simulink model "bd_par_auto2"  (Simulink 4.1.1)
settings: Solver=ode1  SolverMode=SingleTasking  StartTime=0.0  StopTime=max(cyc_mph(:,1))  FixedStep=1  MaxStep=1  RelTol=1e-3  AbsTol=1e-3
undefined symbols (not defined in the file): air_cp, amb_tmp, cs_charge_deplete_bool, cs_charge_trq, cs_electric_decel_spd, cs_electric_launch_spd_hi, cs_electric_launch_spd_lo, cs_hi_soc, cs_lo_soc, cs_min_trq_frac, cs_off_trq_frac, cyc_avg_time, cyc_cargo_mass, cyc_elevation_init, cyc_filter_bool, cyc_grade, cyc_mph, enable_stop, ess_cap_scale, ess_coulombic_eff, ess_init_soc, ess_max_ah_cap, ess_max_volts, ess_min_volts, ess_mod_airflow, ess_mod_cp, ess_mod_init_tmp, ess_module_mass, ess_module_num, ess_on, ess_res_scale_coef, ess_res_scale_fun, ess_set_tmp, ess_th_calc, ess_th_res_off, ess_th_res_on, ess_tmp, ess_voc, ex_calc, fc_ct_trq, fc_emis, fc_inertia, fc_map_spd, fc_max_trq, fc_on, fc_spd_scale, fc_trq_scale, fc_tstat, fd_inertia, fd_loss, fd_ratio, gb_dnshift_load, gb_dnshift_spd, gb_gears_num, gb_inertia, gb_num_init, gb_ratio, gb_shift_delay, gb_spd_scale, gb_trq_scale ... (+56)
libraries: lib_wheel2 x12, lib_accessory2 x3, lib_etc x2, lib_drive_cycle2 x1, lib_interactive x1, lib_drive_cycle x1, lib_exhaust x1, lib_fuel_converter3 x1
(part 2 of 18)

== system bd_par_auto2/<cs> control strategy/Automatic Transmission  Control ==
  Bus Selector1 : BusSelector  OutputSignals=shifting  MuxedOutput=off
  Bus Selector10 : BusSelector  OutputSignals=eta_gb  MuxedOutput=off
  Bus Selector4 : BusSelector  OutputSignals=slip_limited  MuxedOutput=off
  Bus Selector7 : BusSelector  OutputSignals=gb_trq_out_r,gb_spd_out_r  MuxedOutput=off
  Memory : Memory  X0=1  InheritSampleTime=off
      settings: RTWStateStorageClass=Auto
  Mux1 : Mux  Inputs=3
  Mux2 : Mux  Inputs=2
  gearbox control for automatic transmission : Subsystem  TreatAsAtomicUnit=on
      settings: RTWFcnNameOpts=Auto  RTWFileNameOpts=Auto
  tag scope: gbControl=global, htcControl=global
  wires:
  Mux1/1 -> [gbControl], Bus Selector1/1
  gearbox control for automatic transmission/3(gear number) -> Mux1/3  "gear_number"
  gearbox control for automatic transmission/2(shifting) -> Mux1/2  "shifting"
  gearbox control for automatic transmission/1(gear ratio) -> Mux1/1  "gear_ratio"
  Memory/1 -> gearbox control for automatic transmission/1("eta_gb, t=(i-1)")
  [gbReqOut] -> Bus Selector7/1
  Bus Selector7/1 -> gearbox control for automatic transmission/2(T_gb_out)  "<gb_trq_out_r>"
  Bus Selector10/1 -> Memory/1  "<eta_gb>"
  [gbSensors] -> Bus Selector10/1
  [vehReqOut] -> Bus Selector4/1
  Bus Selector4/1 -> gearbox control for automatic transmission/4(slip_limited)  "<slip_limited>"
  Bus Selector7/2 -> gearbox control for automatic transmission/3(w_gb_out)  "<gb_spd_out_r>"
  Mux2/1 -> [htcControl]
  gearbox control for automatic transmission/4(locked_up) -> Mux2/2  "lock_up"
  Bus Selector1/1 -> Mux2/1  "<shifting>"

== system bd_par_auto2/<cs> control strategy/Clutch Control ==
  Bus Creator : BusCreator  Inputs=3
  Bus Selector : BusSelector  OutputSignals=mpha  MuxedOutput=off
  Bus Selector1 : BusSelector  OutputSignals=shifting  MuxedOutput=off
  Bus Selector2 : BusSelector  OutputSignals=gb_spd_in_a  MuxedOutput=off
  Bus Selector3 : BusSelector  OutputSignals=clutch_trq_out_r  MuxedOutput=off
  Bus Selector4 : BusSelector  OutputSignals=clutch_spd_out_r  MuxedOutput=off
  Bus Selector5 : BusSelector  OutputSignals=veh_spd_a_rec  MuxedOutput=off
  Bus Selector6 : BusSelector  OutputSignals=cycle_mph_r  MuxedOutput=off
  Bus Selector7 : BusSelector  OutputSignals=v_ave_req  MuxedOutput=off
  Bus Selector8 : BusSelector  OutputSignals=engine_on  MuxedOutput=off
  Clutch Control : Subsystem  TreatAsAtomicUnit=on
      settings: RTWFcnNameOpts=Auto  RTWFileNameOpts=Auto
  Memory1 : Memory  X0=0  InheritSampleTime=off
      settings: RTWStateStorageClass=Auto
  Memory2 : Memory  X0=cyc_mph(1,2)  InheritSampleTime=off
      settings: RTWStateStorageClass=Auto
  Memory3 : Memory  X0=0  InheritSampleTime=off
      settings: RTWStateStorageClass=Auto
  Memory4 : Memory  X0=cyc_mph(1,2)  InheritSampleTime=off
      settings: RTWStateStorageClass=Auto
  tag scope: clControl=global
  wires:
  Memory4/1 -> Clutch Control/7(cyc_mph_r)
  Memory3/1 -> Clutch Control/6(veh_spd_a_rec)
  Memory2/1 -> Clutch Control/5(mpha)
  Memory1/1 -> Clutch Control/2(gb_spd_in_a)
  Clutch Control/3(launch_flag) -> Bus Creator/3  "launch_flag"
  Bus Selector4/1 -> Clutch Control/4(w_cl_out)  "<clutch_spd_out_r>"
  Bus Selector3/1 -> Clutch Control/3(T_cl_out)  "<clutch_trq_out_r>"
  [clReqOut] -> Bus Selector4/1, Bus Selector3/1
  Bus Selector2/1 -> Memory1/1  "<gb_spd_in_a>"
  [gbSensors] -> Bus Selector2/1
  Bus Selector1/1 -> Clutch Control/1(shifting)  "<shifting>"
  [gbControl] -> Bus Selector1/1
  Clutch Control/2(launch_speed) -> Bus Creator/2  "launch_speed"
  Clutch Control/1(clutch_state) -> Bus Creator/1  "clutch_state"
  Bus Creator/1 -> [clControl]
  [vehSensors] -> Bus Selector/1
  Bus Selector/1 -> Memory2/1  "<mpha>"
  [vehSensors] -> Bus Selector5/1
  Bus Selector5/1 -> Memory3/1  "<veh_spd_a_rec>"
  [cycReqOut] -> Bus Selector6/1
  Bus Selector6/1 -> Memory4/1  "<cycle_mph_r>"
  [vehReqOut] -> Bus Selector7/1
  Bus Selector7/1 -> Clutch Control/8(v_ave_req)  "<v_ave_req>"
  [fcControl] -> Bus Selector8/1
  Bus Selector8/1 -> Clutch Control/9(engine_on?)  "<engine_on>"

== system bd_par_auto2/<cs> control strategy/Drive Cycle ==
  Bus Creator : BusCreator  Inputs=4
  Bus Selector : BusSelector  OutputSignals=mpha  MuxedOutput=off
  Constant : Constant  Value=0
  drive cycle dummy controller : lib_drive_cycle2/drive cycle controls/drive cycle dummy controller
      settings: RTWFcnNameOpts=Auto  RTWFileNameOpts=Auto
  tag scope: cycControl=global
  wires:
  [vehSensors] -> Bus Selector/1
  Bus Selector/1 -> drive cycle dummy controller/1  "<mpha>"
  Constant/1 -> drive cycle dummy controller/3, drive cycle dummy controller/2, drive cycle dummy controller/4
  drive cycle dummy controller/1 -> Bus Creator/1  "mpha"
  drive cycle dummy controller/2 -> Bus Creator/2  "altia_grade"
  drive cycle dummy controller/3 -> Bus Creator/3  "Altia_Run"
  drive cycle dummy controller/4 -> Bus Creator/4  "altia_cyc_mph_r"
  Bus Creator/1 -> [cycControl]

== system bd_par_auto2/<cs> control strategy/Electrical Accessories ==
  Bus Creator : BusCreator  Inputs=4
  Bus Selector1 : BusSelector  OutputSignals=F_req  MuxedOutput=off
  Bus Selector2 : BusSelector  OutputSignals=key_on  MuxedOutput=off
  Bus Selector3 : BusSelector  OutputSignals=engine_on  MuxedOutput=off
  Constant : Constant  Value=ess_on*1
  electrical accessory controller : Subsystem
      settings: RTWFcnNameOpts=Auto  RTWFileNameOpts=Auto
  tag scope: acceControl=global
  wires:
  Constant/1 -> electrical accessory controller/1(electrical accessories on?)
  Bus Creator/1 -> [acceControl]
  [fcControl] -> Bus Selector2/1
  Bus Selector2/1 -> electrical accessory controller/3(key_on in)  "<key_on>"
  [fcControl] -> Bus Selector3/1
  Bus Selector3/1 -> electrical accessory controller/4(engine_on in)  "<engine_on>"
  [vehReqOut] -> Bus Selector1/1
  Bus Selector1/1 -> electrical accessory controller/2(F_req in)  "<F_req>"
  electrical accessory controller/1(acc_on) -> Bus Creator/1
  electrical accessory controller/2(F_req) -> Bus Creator/2
  electrical accessory controller/3(key_on) -> Bus Creator/3
  electrical accessory controller/4(engine_on) -> Bus Creator/4

== system bd_par_auto2/<cs> control strategy/Fuel Converter Control parallel hybrid  ic engine ==
  note: Controls for Fuel Converter:
      | IC Engine for Parallel Hybrid
  Bus Creator : BusCreator  Inputs=10
  Bus Selector1 : BusSelector  OutputSignals=clutch_state  MuxedOutput=off
  Bus Selector10 : BusSelector  OutputSignals=v_req_limited  MuxedOutput=off
  Bus Selector11 : BusSelector  OutputSignals=SOC  MuxedOutput=off
  Bus Selector12 : BusSelector  OutputSignals=ess_max_pwr  MuxedOutput=off
  Bus Selector13 : BusSelector  OutputSignals=fc_clt_tmp  MuxedOutput=off
  Bus Selector14 : BusSelector  OutputSignals=T_cl_out  MuxedOutput=off
  Bus Selector15 : BusSelector  OutputSignals=w_cl_out  MuxedOutput=off
  Bus Selector2 : BusSelector  OutputSignals=shifting  MuxedOutput=off
  Bus Selector3 : BusSelector  OutputSignals=acc_mech_trq_a  MuxedOutput=off
  Bus Selector4 : BusSelector  OutputSignals=v_prev  MuxedOutput=off
  Bus Selector5 : BusSelector  OutputSignals=cycle_mph_r  MuxedOutput=off
  Bus Selector6 : BusSelector  OutputSignals=veh_spd_a_rec  MuxedOutput=off
  Bus Selector7 : BusSelector  OutputSignals=gear_ratio  MuxedOutput=off
  Bus Selector8 : BusSelector  OutputSignals=current_veh_mass  MuxedOutput=off
  Bus Selector9 : BusSelector  OutputSignals=mpha  MuxedOutput=off
  Fuel Converter Control : Subsystem
      settings: RTWFcnNameOpts=Auto  RTWFileNameOpts=Auto
  Memory{1..3,5} (4 alike) : Memory  X0=0  InheritSampleTime=off
      settings: RTWStateStorageClass=Auto
  tag scope: fcControl=global
  wires:
  Bus Selector2/1 -> Fuel Converter Control/9(shifting)  "<shifting>"
  Bus Selector7/1 -> Fuel Converter Control/3(gear_ratio)  "<gear_ratio>"
  Bus Selector1/1 -> Fuel Converter Control/1(clutch_state)  "<clutch_state>"
  [clControl] -> Bus Selector1/1
  [gbControl] -> Bus Selector7/1
  [fcSensors] -> Fuel Converter Control/8(fcSensors)
  [vehReqOut] -> Bus Selector4/1
  Bus Selector4/1 -> Fuel Converter Control/10(v_prev)  "<v_prev>"
  [gbControl] -> Bus Selector2/1
  [accmSensors] -> Bus Selector3/1
  Bus Selector3/1 -> Memory5/1  "<acc_mech_trq_a>"
  Memory5/1 -> Fuel Converter Control/7(acc_mech_trq_est)
  [cycReqOut] -> Bus Selector5/1
  Bus Selector5/1 -> Memory3/1  "<cycle_mph_r>"
  [vehSensors] -> Bus Selector6/1
  Bus Selector6/1 -> Memory2/1  "<veh_spd_a_rec>"
  [cycSensors] -> Bus Selector8/1
  Bus Selector8/1 -> Fuel Converter Control/4(current_veh_mass)  "<current_veh_mass>"
  [vehSensors] -> Bus Selector9/1
  Bus Selector9/1 -> Memory1/1  "<mpha>"
  Fuel Converter Control/10(v_prev out) -> Bus Creator/10  "v_prev"
  Fuel Converter Control/9(key_on out) -> Bus Creator/9  "key_on"
  Fuel Converter Control/8(engine_on out) -> Bus Creator/8  "engine_on"
  Fuel Converter Control/7(acc_mech_trq_est out) -> Bus Creator/7  "acc_mech_trq_est"
  Fuel Converter Control/6(cyc_mph_r out) -> Bus Creator/6  "cyc_mph_r_prev"
  Fuel Converter Control/5(veh spd a rec out) -> Bus Creator/5  "veh_spd_a_rec_prev"
  Fuel Converter Control/4(current veh mass out) -> Bus Creator/4  "current_veh_mass"
  Fuel Converter Control/3(gear_ratio out) -> Bus Creator/3  "gear_ratio"
  Fuel Converter Control/2(miles per hour out) -> Bus Creator/2  "mpha_prev"
  Fuel Converter Control/1(clutch state out) -> Bus Creator/1  "clutch_state"
  Bus Creator/1 -> [fcControl]
  Memory1/1 -> Fuel Converter Control/2(mpha(t-1) (prev))
  Memory2/1 -> Fuel Converter Control/5(veh_spd_a_rec(t-1) (prev))
  Memory3/1 -> Fuel Converter Control/6(cyc_mph_r(t-1) (prev))
  [vehSensors] -> Bus Selector10/1
  Bus Selector10/1 -> Fuel Converter Control/11(v_req_limited)  "<v_req_limited>"
  [essSensors] -> Bus Selector11/1
  Bus Selector11/1 -> Fuel Converter Control/12(SOC)  "<SOC>"
  [essSensors] -> Bus Selector12/1
  Bus Selector12/1 -> Fuel Converter Control/13(ess_max_pwr)  "<ess_max_pwr>"
  [fcSensors] -> Bus Selector13/1
  Bus Selector13/1 -> Fuel Converter Control/14(fc_clt_tmp)  "<fc_clt_tmp>"
  [clSensors] -> Bus Selector14/1
  Bus Selector14/1 -> Fuel Converter Control/15(T_cl_out)  "<T_cl_out>"
  [clSensors] -> Bus Selector15/1
  Bus Selector15/1 -> Fuel Converter Control/16(w_cl_out)  "<w_cl_out>"

== system bd_par_auto2/<cs> control strategy/Hybrid  Engine Torque Modification Strategy ==
  Bus Creator : BusCreator  Inputs=3
  Bus Selector : BusSelector  OutputSignals=tm_spd_out_r  MuxedOutput=off
  Bus Selector1 : BusSelector  OutputSignals=SOC  MuxedOutput=off
  Bus Selector2 : BusSelector  OutputSignals=engine_on  MuxedOutput=off
  parallel auto hybrid torque control : Subsystem
      settings: RTWFcnNameOpts=Auto  RTWFileNameOpts=Auto
  tag scope: tmControl=global
  wires:
  parallel auto hybrid torque control/1(tm_torqueMod) -> Bus Creator/1  "tm_torqueMod"
  parallel auto hybrid torque control/2(tm_torqueMin) -> Bus Creator/2  "tm_torqueMin"
  parallel auto hybrid torque control/3(tm_enable) -> Bus Creator/3  "tm_enable"
  Bus Creator/1 -> [tmControl]
  [tmReqOut] -> Bus Selector/1
  Bus Selector/1 -> parallel auto hybrid torque control/1(tm_spd_out_r)  "<tm_spd_out_r>"
  [essSensors] -> Bus Selector1/1
  Bus Selector1/1 -> parallel auto hybrid torque control/2(SOC)  "<SOC>"
  [fcControl] -> Bus Selector2/1
  Bus Selector2/1 -> parallel auto hybrid torque control/3(engine_on)  "<engine_on>"

== system bd_par_auto2/<cs> control strategy/Mechanical Accessories ==
  Bus Creator : BusCreator  Inputs=9
  Bus Selector : BusSelector  OutputSignals=fc_spd_est  MuxedOutput=off
  Bus Selector1 : BusSelector  OutputSignals=F_req  MuxedOutput=off
  Bus Selector2 : BusSelector  OutputSignals=key_on  MuxedOutput=off
  Bus Selector3 : BusSelector  OutputSignals=engine_on  MuxedOutput=off
  Constant : Constant  Value=not(ess_on)*1
  Constant1 : Constant  Value=inf
  Constant2 : Constant  Value=(vc_idle_spd*vc_idle_bool)+eps
  mechanical accessory controller : Subsystem
      settings: RTWFcnNameOpts=Auto  RTWFileNameOpts=Auto
  tag scope: accmControl=global
  wires:
  Constant1/1 -> mechanical accessory controller/2(maximum accessory speed)
  Constant2/1 -> mechanical accessory controller/3(minimum accessory speed)
  Constant/1 -> mechanical accessory controller/4(electrical accessories on?)
  mechanical accessory controller/1(acc_on) -> Bus Creator/1
  mechanical accessory controller/2(acc_mech_spd_r) -> Bus Creator/2
  mechanical accessory controller/3(acc_mech_spd_a) -> Bus Creator/3
  mechanical accessory controller/4(acc_max_spd) -> Bus Creator/4
  mechanical accessory controller/5(acc_min_spd) -> Bus Creator/5
  mechanical accessory controller/6(elec_acc_on_bool) -> Bus Creator/6
  mechanical accessory controller/7(F_req) -> Bus Creator/7
  mechanical accessory controller/8(key_on) -> Bus Creator/8
  mechanical accessory controller/9(engine_on) -> Bus Creator/9
  Bus Creator/1 -> [accmControl]
  [fcControl] -> Bus Selector2/1
  Bus Selector2/1 -> mechanical accessory controller/6(key on?)  "<key_on>"
  [fcControl] -> Bus Selector3/1
  Bus Selector3/1 -> mechanical accessory controller/7(engine on?)  "<engine_on>"
  [fcReqOut] -> Bus Selector/1
  Bus Selector/1 -> mechanical accessory controller/1(accessory reference shaft speed)  "<fc_spd_est>"
  [vehReqOut] -> Bus Selector1/1
  Bus Selector1/1 -> mechanical accessory controller/5(Force required for vehicle motion)  "<F_req>"

== system bd_par_auto2/<cs> control strategy/Motor Controller ==
  Bus Selector : BusSelector  OutputSignals=v_prev  MuxedOutput=off
  Bus Selector1 : BusSelector  OutputSignals=key_on  MuxedOutput=off
  Bus Selector2 : BusSelector  OutputSignals=veh_spd_a_rec  MuxedOutput=off
  Bus Selector3 : BusSelector  OutputSignals=bus_voltage  MuxedOutput=off
  Bus Selector4 : BusSelector  OutputSignals=mpha  MuxedOutput=off
  Bus Selector5 : BusSelector  OutputSignals=cycle_mph_r  MuxedOutput=off
  Bus Selector6 : BusSelector  OutputSignals=current_veh_mass  MuxedOutput=off
  Bus Selector7 : BusSelector  OutputSignals=shifting  MuxedOutput=off
  Constant : Constant  Value=cyc_mph(1,2)*0.447/wh_radius*fd_ratio*max(gb_ratio)*tc_mc_to_fc_ratio
  Memory{,1..3} (4 alike) : Memory  X0=ess_module_num*mean(ess_voc(1,:))  InheritSampleTime=off
      settings: RTWStateStorageClass=Auto
  Mux : Mux  Inputs=9
  motor controller : Subsystem
      settings: RTWFcnNameOpts=Auto  RTWFileNameOpts=Auto
  tag scope: mcControl=global
  wires:
  [vehSensors] -> Bus Selector/1
  Bus Selector/1 -> motor controller/1(v_prev in)  "<v_prev>"
  [fcControl] -> Bus Selector1/1
  Bus Selector1/1 -> motor controller/2(key_on in)  "<key_on>"
  [vehSensors] -> Bus Selector2/1
  Bus Selector2/1 -> Memory3/1  "<veh_spd_a_rec>"
  [essSensors] -> Bus Selector3/1
  Bus Selector3/1 -> Memory/1  "<bus_voltage>"
  Memory/1 -> motor controller/4(bus voltage previous)
  [vehSensors] -> Bus Selector4/1
  Bus Selector4/1 -> Memory1/1  "<mpha>"
  [cycReqOut] -> Bus Selector5/1
  Bus Selector5/1 -> Memory2/1  "<cycle_mph_r>"
  [cycSensors] -> Bus Selector6/1
  Bus Selector6/1 -> motor controller/7(current vehicle mass)  "<current_veh_mass>"
  [gbControl] -> Bus Selector7/1
  Bus Selector7/1 -> motor controller/8(shifting)  "<shifting>"
  motor controller/1(v_prev) -> Mux/1  "v_prev"
  motor controller/2(key_on) -> Mux/2  "key_on"
  motor controller/3(veh_spd_a_rec_prev out) -> Mux/3  "veh_spd_a_rec_prev"
  motor controller/4(bus_voltage_prev) -> Mux/4  "bus_voltage_prev"
  motor controller/5(mpha_prev out) -> Mux/5  "mpha_prev"
  motor controller/6(cyc_mph_r_prev) -> Mux/6  "cyc_mph_r_prev"
  motor controller/7(current_veh_mass) -> Mux/7  "current_veh_mass"
  motor controller/8(shifting out) -> Mux/8  "shifting"
  Mux/1 -> [mcControl]
  Memory1/1 -> motor controller/5(mpha_prev in)
  Memory2/1 -> motor controller/6(cyc_mph_r_prev in)
  Memory3/1 -> motor controller/3(veh_spd_a_rec_prev in)
  Constant/1 -> motor controller/9(mc_spd_init_est in)
  motor controller/9(mc_spd_init_est out) -> Mux/9  "mc_spd_init_est"

== system bd_par_auto2/<cs> control strategy/Power Bus ==
  Constant : Constant  Value=ess_on*1
  power bus controller : Subsystem
      settings: RTWFcnNameOpts=Auto  RTWFileNameOpts=Auto
  tag scope: pbControl=global
  wires:
  power bus controller/1(ess_on) -> [pbControl]
  Constant/1 -> power bus controller/1(enable source two on power bus?)

== system bd_par_auto2/<cs> control strategy/Wheel Control ==
  Bus Selector : BusSelector  OutputSignals=v_init  MuxedOutput=off
  Bus Selector1 : BusSelector  OutputSignals=current_veh_mass  MuxedOutput=off
  Bus Selector2 : BusSelector  OutputSignals=grade  MuxedOutput=off
  dummy controls : lib_wheel2/vehicle controls/dummy controls
      settings: RTWFcnNameOpts=Auto  RTWFileNameOpts=Auto
  tag scope: vehControl=global
  wires:
  [cycReqOut] -> Bus Selector/1
  Bus Selector/1 -> dummy controls/1  "<v_init>"
  Bus Selector1/1 -> dummy controls/2  "<current_veh_mass>"
  Bus Selector2/1 -> dummy controls/3  "<grade>"
  [cycSensors] -> Bus Selector2/1
  [cycSensors] -> Bus Selector1/1
  dummy controls/1 -> [vehControl]

== system bd_par_auto2/ACC MECH <accm>/mechanical accessory model and interface ==
  note: w_APU_speed is the reference speed for accessories requiring a speed lookup
      | it may be different from acc_mech_spd_r if that value was limited by acc_max_spd
      | or acc_min_spd
  note: * elec_acc_on_bool Enables/Disables electrical accessories only-- it was originally conceived as a means to have electrical accessory loads be
      | satisfieed by either a mechanical generator or an electrical power bus
      |
      | F_req is the force required by the wheels for traction power (used as a trigger for brake light accessories)
      |
      | key_on is used as a trigger for some electrical accessories (indicates if the vehicle is "powered on" or not
      |
      | engine_on is used as a trigger for some electrical accessories (indicates whether the internal combustion engine is running or not) used
      | for starter motor
  note: *
  note: Enables/Disables the entire accessory system
  note: INTERFACE
  "T, w out requested" : Inport  Port=1  LatchInput=off
  "T, w in achieved" : Inport  Port=2  LatchInput=off
  control : Inport  Port=3  LatchInput=off
  Block NOTES : Subsystem
      settings: RTWFcnNameOpts=Auto  RTWFileNameOpts=Auto
      mask Display: disp('Block\nNOTES')
  Bus Creator : BusCreator  Inputs=5
  Demux : Demux  Outputs=9  BusSelectionMode=off
  Goto Tag Visibility1 : GotoTagVisibility  GotoTag=acc_mech_spd_r
  Goto Tag Visibility10 : GotoTagVisibility  GotoTag=acc_min_spd
  Goto Tag Visibility11 : GotoTagVisibility  GotoTag=F_req
  Goto Tag Visibility12 : GotoTagVisibility  GotoTag=key_on
  Goto Tag Visibility13 : GotoTagVisibility  GotoTag=engine_on
  Goto Tag Visibility14 : GotoTagVisibility  GotoTag=w_APU_speed
  Goto Tag Visibility2 : GotoTagVisibility  GotoTag=acc_mech_pwr_a
  Goto Tag Visibility3 : GotoTagVisibility  GotoTag=acc_mech_trq_a
  Goto Tag Visibility4 : GotoTagVisibility  GotoTag=acc_mech_spd_a
  Goto Tag Visibility5 : GotoTagVisibility  GotoTag=acc_mech_trq_r
  Goto Tag Visibility6 : GotoTagVisibility  GotoTag=acc_mech_pwr_r
  Goto Tag Visibility7 : GotoTagVisibility  GotoTag=elec_acc_on_bool
  Goto Tag Visibility8 : GotoTagVisibility  GotoTag=acc_max_spd
  Goto Tag Visibility9 : GotoTagVisibility  GotoTag=acc_on
  Mechanical Accessory model : Subsystem
      settings: RTWFcnNameOpts=Auto  RTWFileNameOpts=Auto
      mask Display: image(imread('bdi_acc_pic.bmp'))
  help : Subsystem
      settings: OpenFcn=web(['file:\\\' which('motor_controller.htm')]);  RTWFcnNameOpts=Auto  RTWFileNameOpts=Auto
      mask Display: image(imread('doc_man.jpg'))
  signal annotator : Subsystem
      settings: RTWFcnNameOpts=Auto  RTWFileNameOpts=Auto
  Out Request : Outport  Port=1
  T,w in request : Outport  Port=2
  "T, w out achieved" : Outport  Port=3
  sensors : Outport  Port=4
  tag scope: F_req=scoped, acc_max_spd=scoped, acc_mech_spd_a=scoped, acc_mech_spd_r=scoped, acc_min_spd=scoped, acc_on=scoped, elec_acc_on_bool=scoped, engine_on=scoped, key_on=scoped
  wires:
  Demux/9 -> [engine_on]
  Demux/8 -> [key_on]
  Demux/7 -> [F_req]
  [w_APU_speed] -> Bus Creator/5  "w_APU_speed"
  Demux/6 -> [elec_acc_on_bool]
  signal annotator/1(Out1) -> Out Request/1
  control/1 -> Demux/1
  Bus Creator/1 -> sensors/1
  Demux/5 -> [acc_min_spd]
  Demux/4 -> [acc_max_spd]
  Demux/3 -> [acc_mech_spd_a]
  [acc_mech_pwr_r] -> Bus Creator/4  "acc_mech_pwr_r"
  [acc_mech_trq_r] -> Bus Creator/3  "acc_mech_trq_r"
  [acc_mech_pwr_a] -> Bus Creator/2  "acc_mech_pwr_a"
  [acc_mech_trq_a] -> Bus Creator/1  "acc_mech_trq_a"
  Demux/2 -> [acc_mech_spd_r]
  Demux/1 -> [acc_on]
  Mechanical Accessory model/2("achieved shaft T and w, out to the driveline (Nm ; rad/s)") -> "T, w out achieved"/1
  "T, w in achieved"/1 -> Mechanical Accessory model/2("achieved shaft and belt T and w, in from the prime mover (Nm ; rad/s)")
  Mechanical Accessory model/1("requested shaft and belt T and w, in from the prime mover (Nm ; rad/s)") -> T,w in request/1
  "T, w out requested"/1 -> signal annotator/1(In1), Mechanical Accessory model/1("requested shaft T and w, out to the driveline  (Nm ; rad/s; rad/s)")

== system bd_par_auto2/NOTES/NOTES ==
  note: ADVISOR 2.0.2 10/7/98
      | Copyright 1998-2003  MRI, NREL.
      | All rights reserved
      |
      |  Notice:  This computer software was
      |  prepared by NREL/MRI, and hereinafter the Contractor,
      | under Contract No. DE-AC36-83CH10093 with
      | the Department of Energy (DOE).  All rights
      | in the computer software are reserved by DOE
      | on behalf of the United States Government and
      | the Contractor as provided in the contract.
      | You are authorized to use this computer software
      | for Governmental purposes but it is not to be
      | released or distributed to the public.  NEITHER
      | THE GOVERNMENT NOR THE CONTRACTOR MAKES ANY
      | WARRANTY, EXPRESS OR IMPLIED, OR ASSUMES ANY
      | LIABILITY FOR THE USE OF THIS SOFTWARE.
      | This notice including this sentence must
      | appear on any copies of this computer software.

== system bd_par_auto2/clutch <cl>/clutch model and interface ==
  note: Model
  note: Interface
  T & w output requested : Inport  Port=1  LatchInput=off
  T & w input achieved : Inport  Port=2  LatchInput=off
  control : Inport  Port=3  LatchInput=off
  Bus Creator : BusCreator  Inputs=2
  Demux2 : Demux  Outputs=3  BusSelectionMode=off
  Goto Tag Visibility : GotoTagVisibility  GotoTag=clutch_state
  Goto Tag Visibility1 : GotoTagVisibility  GotoTag=T_cl_out
  Goto Tag Visibility2 : GotoTagVisibility  GotoTag=w_cl_out
  Goto Tag Visibility3 : GotoTagVisibility  GotoTag=launch_speed
  Goto Tag Visibility4 : GotoTagVisibility  GotoTag=launch_flag
  clutch model : Subsystem
      settings: RTWFcnNameOpts=Auto  RTWFileNameOpts=Auto
  signal annotator : Subsystem
      settings: RTWFcnNameOpts=Auto  RTWFileNameOpts=Auto
  required out : Outport  Port=1
  Out1 : Outport  Port=2
  Out2 : Outport  Port=3
  sensors : Outport  Port=4
  tag scope: clutch_state=scoped, launch_flag=scoped, launch_speed=scoped
  wires:
  signal annotator/1(Out1) -> required out/1
  Bus Creator/1 -> sensors/1
  clutch model/2(T & w output achieved) -> Out2/1
  T & w input achieved/1 -> clutch model/2(T & w input achieved)
  clutch model/1(T & w input request) -> Out1/1
  T & w output requested/1 -> signal annotator/1(In1), clutch model/1(T & w output requested)
  [w_cl_out] -> Bus Creator/2  "w_cl_out"
  [T_cl_out] -> Bus Creator/1  "T_cl_out"
  Demux2/3 -> [launch_flag]
  Demux2/2 -> [launch_speed]
  Demux2/1 -> [clutch_state]
  control/1 -> Demux2/1

== system bd_par_auto2/drive cycle <cyc>/drive cycle model and interface ==
  note: DRIVE CYCLE
      | interface
  note: DRIVE CYCLE
      | model
  control : Inport  Port=1  LatchInput=off
  Bus Creator : BusCreator  Inputs=5
  Clock : Clock
      settings: DisplayTime=off  Decimation=10
  Constant : Constant  Value=veh_mass
  Demux : Demux  Outputs=4  BusSelectionMode=off
  Goto Tag Visibility : GotoTagVisibility  GotoTag=mpha
  Goto Tag Visibility1 : GotoTagVisibility  GotoTag=distance
  Goto Tag Visibility10 : GotoTagVisibility  GotoTag=altia_cyc_mph_r
  Goto Tag Visibility2 : GotoTagVisibility  GotoTag=grade_orig
  Goto Tag Visibility3 : GotoTagVisibility  GotoTag=altia_grade
  Goto Tag Visibility4 : GotoTagVisibility  GotoTag=Altia_Run
  Goto Tag Visibility5 : GotoTagVisibility  GotoTag=grade
  Goto Tag Visibility6 : GotoTagVisibility  GotoTag=elevation
  Goto Tag Visibility7 : GotoTagVisibility  GotoTag=veh_cargo_mass
  Goto Tag Visibility8 : GotoTagVisibility  GotoTag=cyc_mph_r_orig
  Goto Tag Visibility9 : GotoTagVisibility  GotoTag=cyc_mph_r
  Sum : Sum  Inputs=++|  SaturateOnIntegerOverflow=on
  drive cycle model : Subsystem
      settings: RTWFcnNameOpts=Auto  RTWFileNameOpts=Auto
  signal annotator : Subsystem
      settings: RTWFcnNameOpts=Auto  RTWFileNameOpts=Auto
  req'd lookups : Outport  Port=1  InitialOutput=0
  req'd vehicle speed (m/s) : Outport  Port=2  InitialOutput=0
  sensors : Outport  Port=3  InitialOutput=0
  tag scope: Altia_Run=scoped, altia_cyc_mph_r=scoped, altia_grade=scoped, mpha=scoped
  wires:
  Sum/1 -> Bus Creator/5  "current_veh_mass"
  Constant/1 -> Sum/2
  [cyc_mph_r] -> signal annotator/3(In3)  "cyc_mph_r"
  [cyc_mph_r_orig] -> signal annotator/2(In2)  "cyc_mph_r_orig"
  [veh_cargo_mass] -> Sum/1  "veh_cargo_mass"
  [elevation] -> Bus Creator/4  "elevation"
  [grade] -> Bus Creator/3  "grade"
  [grade_orig] -> Bus Creator/2  "grade_orig"
  [distance] -> Bus Creator/1  "distance"
  Demux/4 -> [altia_cyc_mph_r]
  Demux/3 -> [Altia_Run]
  Demux/2 -> [altia_grade]
  Demux/1 -> [mpha]
  Bus Creator/1 -> sensors/1
  control/1 -> Demux/1
  signal annotator/1(Out1) -> req'd lookups/1
  Clock/1 -> signal annotator/1(In1)
  drive cycle model/1(req'd vehicle speed (m/s)) -> req'd vehicle speed (m/s)/1

== system bd_par_auto2/ess config/energy storage <ess> ==
  note: Energy Storage System
  power req'd into bus (W) : Inport  Port=1  LatchInput=off
  Block NOTES : Subsystem
      settings: RTWFcnNameOpts=Auto  RTWFileNameOpts=Auto
      mask Display: disp('Block\nNOTES')
  documentation9 : Subsystem
      settings: OpenFcn=web(['file:\\\' which('energy_storage.htm')]);  RTWFcnNameOpts=Auto  RTWFileNameOpts=Auto
      mask Display: image(imread('doc_man.jpg'))
  energy storage <ess> : Subsystem
      settings: RTWFcnNameOpts=Auto  RTWFileNameOpts=Auto
      mask Display: image(imread('bdi_ess.jpg'))
  power available to bus (W) : Outport  Port=1  InitialOutput=0
  tag scope: essReqOut=global, essSensors=global
  wires:
  energy storage <ess>/3(sensors) -> [essSensors]
  energy storage <ess>/2(power available to bus (W)) -> power available to bus (W)/1
  energy storage <ess>/1(required out) -> [essReqOut]
  [essControl] -> energy storage <ess>/2(control)
  power req'd into bus (W)/1 -> energy storage <ess>/1(power req'd into bus (W))

== system bd_par_auto2/final drive <fd>/Block NOTES ==
  note: The inertia torque is the input torque required to accelerate the
      | final drive's inertia as measured on the input side.
  note: The loss torque is zero when the gears are not turning,
      | and is applied at the input side of the gear reduction.
  note: This final drive model includes loss data, rotational inertia, and a gear reduction.

== system bd_par_auto2/final drive <fd>/help ==

== system bd_par_auto2/final drive <fd>/model&interface ==
  note: Model
  note: Interface
  T & w output request : Inport  Port=1  LatchInput=off
  T & w input achieved : Inport  Port=2  LatchInput=off
  control : Inport  Port=3  LatchInput=off
  Ground : Ground
  Terminator : Terminator
  model : Subsystem
      settings: RTWFcnNameOpts=Auto  RTWFileNameOpts=Auto
  signal annotator : Subsystem
      settings: RTWFcnNameOpts=Auto  RTWFileNameOpts=Auto
  out request : Outport  Port=1  InitialOutput=0
  T & w input request : Outport  Port=2  InitialOutput=0
  T & w output achieved : Outport  Port=3  InitialOutput=0
  sensors : Outport  Port=4  InitialOutput=0
  wires:
  signal annotator/1(Out1) -> out request/1
  control/1 -> Terminator/1
  Ground/1 -> sensors/1
  model/2("torque and speed avail. at output side of final drive (Nm), (rad/s)") -> T & w output achieved/1
  T & w input achieved/1 -> model/2("torque and speed avail. at input side of final drive (Nm), (rad/s)")
  T & w output request/1 -> signal annotator/1(In1), model/1("torque and speed req'd at output side of final drive (Nm), (rad/s)")
  model/1("torque and speed req'd at input side of final drive (Nm), (rad/s)") -> T & w input request/1

== system bd_par_auto2/fuel converter <fc>/Block NOTES ==
  note: This block models the internal combustion engine, and includes inertia effects,
      | performance limits, accessory loads, and temperature transient effects on fuel
      | use, engine-out emissions, and catalyst efficiency.  There are 'leads' to the
      | engine controller here, which controller determines whether the engine is on.

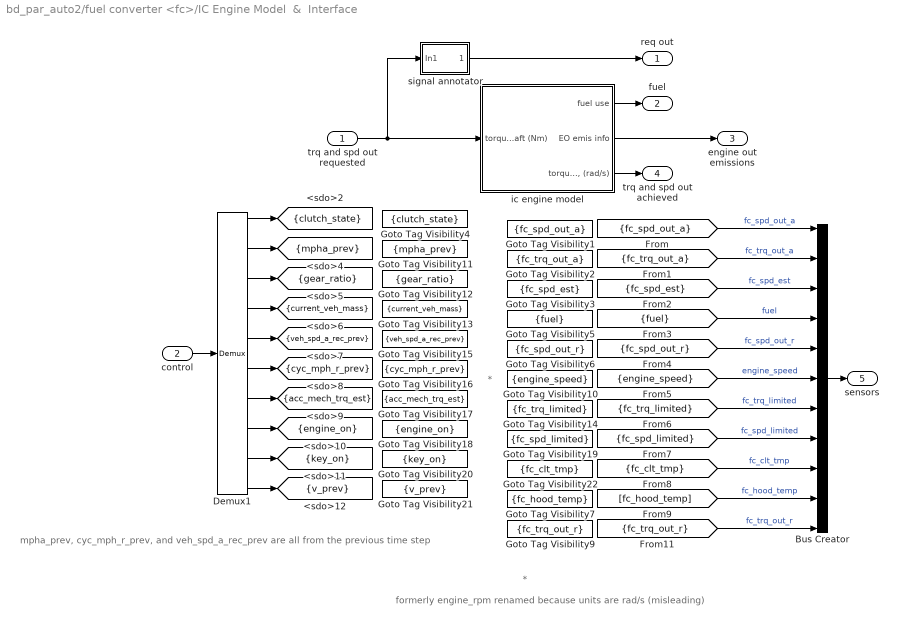
== system bd_par_auto2/fuel converter <fc>/IC Engine Model  &  Interface ==
  note: formerly
      | engine_rpm
      | renamed because
      | units are rad/s
      |  (misleading)
  note: *
  note: *
  note: mpha_prev, cyc_mph_r_prev, and veh_spd_a_rec_prev
      | are all from the previous time step
  trq and spd out requested : Inport  Port=1  LatchInput=off
  control : Inport  Port=2  LatchInput=off
  Bus Creator : BusCreator  Inputs=11
  Demux1 : Demux  Outputs=10  BusSelectionMode=off
  Goto Tag Visibility1 : GotoTagVisibility  GotoTag=fc_spd_out_a
  Goto Tag Visibility10 : GotoTagVisibility  GotoTag=engine_speed
  Goto Tag Visibility11 : GotoTagVisibility  GotoTag=mpha_prev
  Goto Tag Visibility12 : GotoTagVisibility  GotoTag=gear_ratio
  Goto Tag Visibility13 : GotoTagVisibility  GotoTag=current_veh_mass
  Goto Tag Visibility14 : GotoTagVisibility  GotoTag=fc_trq_limited
  Goto Tag Visibility15 : GotoTagVisibility  GotoTag=veh_spd_a_rec_prev
  Goto Tag Visibility16 : GotoTagVisibility  GotoTag=cyc_mph_r_prev
  Goto Tag Visibility17 : GotoTagVisibility  GotoTag=acc_mech_trq_est
  Goto Tag Visibility18 : GotoTagVisibility  GotoTag=engine_on
  Goto Tag Visibility19 : GotoTagVisibility  GotoTag=fc_spd_limited
  Goto Tag Visibility2 : GotoTagVisibility  GotoTag=fc_trq_out_a
  Goto Tag Visibility20 : GotoTagVisibility  GotoTag=key_on
  Goto Tag Visibility21 : GotoTagVisibility  GotoTag=v_prev
  Goto Tag Visibility22 : GotoTagVisibility  GotoTag=fc_clt_tmp
  Goto Tag Visibility3 : GotoTagVisibility  GotoTag=fc_spd_est
  Goto Tag Visibility4 : GotoTagVisibility  GotoTag=clutch_state
  Goto Tag Visibility5 : GotoTagVisibility  GotoTag=fuel
  Goto Tag Visibility6 : GotoTagVisibility  GotoTag=fc_spd_out_r
  Goto Tag Visibility7 : GotoTagVisibility  GotoTag=fc_hood_temp
  Goto Tag Visibility9 : GotoTagVisibility  GotoTag=fc_trq_out_r
  ic engine model : Subsystem
      settings: RTWFcnNameOpts=Auto  RTWFileNameOpts=Auto
  signal annotator : Subsystem
      settings: RTWFcnNameOpts=Auto  RTWFileNameOpts=Auto
  req out : Outport  Port=1
  fuel : Outport  Port=2
  engine out emissions : Outport  Port=3
  trq and spd out achieved : Outport  Port=4
  sensors : Outport  Port=5
  tag scope: acc_mech_trq_est=scoped, clutch_state=scoped, current_veh_mass=scoped, cyc_mph_r_prev=scoped, engine_on=scoped, gear_ratio=scoped, key_on=scoped, mpha_prev=scoped, v_prev=scoped, veh_spd_a_rec_prev=scoped
  wires:
  signal annotator/1(Out1) -> req out/1
  Bus Creator/1 -> sensors/1
  control/1 -> Demux1/1
  ic engine model/3("torque and speed  avail. to driveline (Nm), (rad/s)") -> trq and spd out achieved/1
  ic engine model/2(EO emis info) -> engine out emissions/1
  ic engine model/1(fuel use) -> fuel/1
  trq and spd out requested/1 -> signal annotator/1(In1), ic engine model/1(torque and speed  req'd at engine  output shaft (Nm))
  Demux1/10 -> [v_prev]
  Demux1/9 -> [key_on]
  Demux1/8 -> [engine_on]
  Demux1/7 -> [acc_mech_trq_est]
  Demux1/6 -> [cyc_mph_r_prev]
  Demux1/5 -> [veh_spd_a_rec_prev]
  Demux1/4 -> [current_veh_mass]
  Demux1/3 -> [gear_ratio]
  Demux1/2 -> [mpha_prev]
  Demux1/1 -> [clutch_state]
  [fc_spd_out_a] -> Bus Creator/1  "fc_spd_out_a"
  [fc_trq_out_a] -> Bus Creator/2  "fc_trq_out_a"
  [fc_spd_est] -> Bus Creator/3  "fc_spd_est"
  [fuel] -> Bus Creator/4  "fuel"
  [fc_spd_out_r] -> Bus Creator/5  "fc_spd_out_r"
  [engine_speed] -> Bus Creator/6  "engine_speed"
  [fc_trq_limited] -> Bus Creator/7  "fc_trq_limited"
  [fc_spd_limited] -> Bus Creator/8  "fc_spd_limited"
  [fc_clt_tmp] -> Bus Creator/9  "fc_clt_tmp"
  [fc_hood_temp] -> Bus Creator/10  "fc_hood_temp"
  [fc_trq_out_r] -> Bus Creator/11  "fc_trq_out_r"

== system bd_par_auto2/fuel converter <fc>/help ==

== system bd_par_auto2/gearbox <gb> old/Block NOTES ==
  note: This is a good assumption, at least for the VW 4-speed manual transaxle of SAE 820741.
      | In the VW transaxle, efficiency is fairly independent of torque and speed at high torques.
  note: Available output torque is estimated assuming that the gearbox efficiency for theavailable input
      | torque andspeed is the same as the gearbox efficiency for the REQUESTED input torque.
  note: The inertia torque is the input torque required to accelerate the
      | final drive's inertia as measured on the input side.
  note: The loss torque is zero when the gears are not turning,
      | and is applied at the input side of the gear reduction.
  note: This gearbox model includes loss data, rotational inertia, and a gear reduction.

== system bd_par_auto2/gearbox <gb> old/gearbox model & interface ==
  note: Interface
  note: Model
  trq and spd output request : Inport  Port=1  LatchInput=off
  trq and spd input achieved : Inport  Port=2  LatchInput=off
  controls : Inport  Port=3  LatchInput=off
  Bus Creator : BusCreator  Inputs=5
  Demux2 : Demux  Outputs=3  BusSelectionMode=off
  Goto Tag Visibility : GotoTagVisibility  GotoTag=gear_number
  Goto Tag Visibility1 : GotoTagVisibility  GotoTag=gb_spd_in_a
  Goto Tag Visibility2 : GotoTagVisibility  GotoTag=gear_ratio
  Goto Tag Visibility3 : GotoTagVisibility  GotoTag=shifting
  Goto Tag Visibility4 : GotoTagVisibility  GotoTag=T_gb_out
  Goto Tag Visibility5 : GotoTagVisibility  GotoTag=w_gb_out
  Goto Tag Visibility6 : GotoTagVisibility  GotoTag=eta_gb
  Goto Tag Visibility7 : GotoTagVisibility  GotoTag=gb_trq_out_a
  gearbox model : Subsystem
      settings: RTWFcnNameOpts=Auto  RTWFileNameOpts=Auto
  signal annotator : Subsystem
      settings: RTWFcnNameOpts=Auto  RTWFileNameOpts=Auto
  requested output : Outport  Port=1
  trq and spd input request : Outport  Port=2
  trq and spd output achieved : Outport  Port=3
  sensors : Outport  Port=4
  tag scope: gear_number=scoped, gear_ratio=scoped, shifting=scoped
  wires:
  [gb_trq_out_a] -> Bus Creator/5  "gb_trq_out_a"
  signal annotator/1(Out1) -> requested output/1
  gearbox model/2("torque and speed avail. at output side of gearbox (Nm), (rad/s)") -> trq and spd output achieved/1
  trq and spd input achieved/1 -> gearbox model/2("torque and speed avail. at input side of gearbox (Nm), (rad/s)")
  gearbox model/1("torque and speed req'd at input side of gearbox (Nm), (rad/s)") -> trq and spd input request/1
  trq and spd output request/1 -> signal annotator/1(In1), gearbox model/1("torque and speed req'd at output side of gearbox (Nm), (rad/s)")
  Demux2/3 -> [gear_number]
  Demux2/2 -> [shifting]
  Demux2/1 -> [gear_ratio]
  controls/1 -> Demux2/1
  Bus Creator/1 -> sensors/1
  [eta_gb] -> Bus Creator/4  "eta_gb"
  [w_gb_out] -> Bus Creator/3  "w_gb_out"
  [T_gb_out] -> Bus Creator/2  "T_gb_out"
  [gb_spd_in_a] -> Bus Creator/1  "gb_spd_in_a"

== system bd_par_auto2/gearbox <gb> old/help ==

== system bd_par_auto2/hydraulic torque converter <htc> HEV/HTC for parallel HEV and Interface ==
  note: Interface
  note: Model
  trq and spd output request : Inport  Port=1  LatchInput=off
  trq and spd input achieved : Inport  Port=2  LatchInput=off
  control : Inport  Port=3  LatchInput=off
  Demux : Demux  Outputs=2  BusSelectionMode=off
  Goto Tag Visibility : GotoTagVisibility  GotoTag=shifting
  Goto Tag Visibility2 : GotoTagVisibility  GotoTag=locked_up
  Ground : Ground
  model for parallel HEV : Subsystem
      settings: RTWFcnNameOpts=Auto  RTWFileNameOpts=Auto
  signal annotator : Subsystem
      settings: RTWFcnNameOpts=Auto  RTWFileNameOpts=Auto
  requested output : Outport  Port=1  InitialOutput=0
  trq and spd input request : Outport  Port=2  InitialOutput=0
  trq and spd output achieved : Outport  Port=3  InitialOutput=0
  sensors : Outport  Port=4  InitialOutput=0
  tag scope: locked_up=scoped, shifting=scoped
  wires:
  Ground/1 -> sensors/1
  Demux/2 -> [locked_up]
  Demux/1 -> [shifting]
  control/1 -> Demux/1
  signal annotator/1(Out1) -> requested output/1
  trq and spd input achieved/1 -> model for parallel HEV/2("trq and spd available at input (Nm), (rad/s)")
  model for parallel HEV/2("trq and spd available at output (Nm), (rad/s)") -> trq and spd output achieved/1
  model for parallel HEV/1("req'd input trq and spd (Nm), (rad/s)") -> trq and spd input request/1
  trq and spd output request/1 -> model for parallel HEV/1("req'd output trq and spd (Nm), (rad/s)"), signal annotator/1(In1)

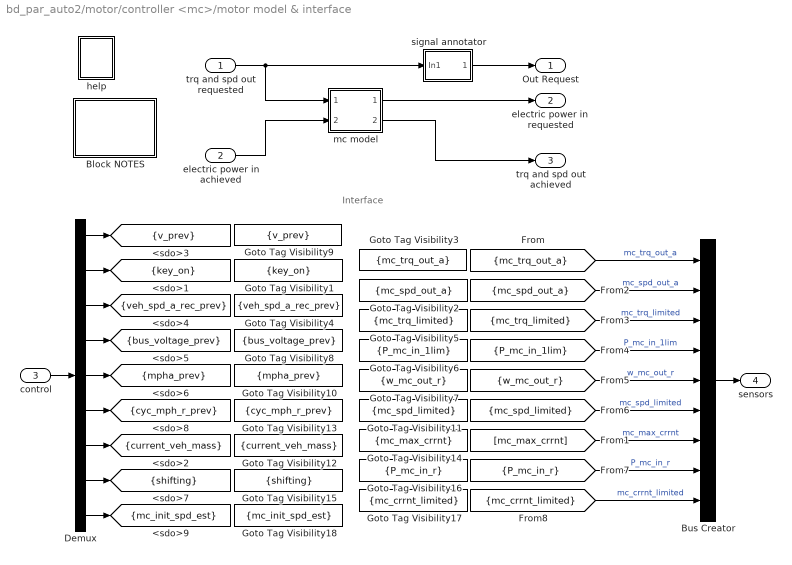
== system bd_par_auto2/motor/controller <mc>/motor model & interface ==
  note: Interface
  trq and spd out requested : Inport  Port=1  LatchInput=off
  electric power in achieved : Inport  Port=2  LatchInput=off
  control : Inport  Port=3  LatchInput=off
  Block NOTES : Subsystem
      settings: RTWFcnNameOpts=Auto  RTWFileNameOpts=Auto
      mask Display: disp('Block\nNOTES')
  Bus Creator : BusCreator  Inputs=9
  Demux : Demux  Outputs=9  BusSelectionMode=off
  Goto Tag Visibility1 : GotoTagVisibility  GotoTag=key_on
  Goto Tag Visibility10 : GotoTagVisibility  GotoTag=mpha_prev
  Goto Tag Visibility11 : GotoTagVisibility  GotoTag=mc_spd_limited
  Goto Tag Visibility12 : GotoTagVisibility  GotoTag=current_veh_mass
  Goto Tag Visibility13 : GotoTagVisibility  GotoTag=cyc_mph_r_prev
  Goto Tag Visibility14 : GotoTagVisibility  GotoTag=mc_max_crrnt
  Goto Tag Visibility15 : GotoTagVisibility  GotoTag=shifting
  Goto Tag Visibility16 : GotoTagVisibility  GotoTag=P_mc_in_r
  Goto Tag Visibility17 : GotoTagVisibility  GotoTag=mc_crrnt_limited
  Goto Tag Visibility18 : GotoTagVisibility  GotoTag=mc_init_spd_est
  Goto Tag Visibility2 : GotoTagVisibility  GotoTag=mc_spd_out_a
  Goto Tag Visibility3 : GotoTagVisibility  GotoTag=mc_trq_out_a
  Goto Tag Visibility4 : GotoTagVisibility  GotoTag=veh_spd_a_rec_prev
  Goto Tag Visibility5 : GotoTagVisibility  GotoTag=mc_trq_limited
  Goto Tag Visibility6 : GotoTagVisibility  GotoTag=P_mc_in_1lim
  Goto Tag Visibility7 : GotoTagVisibility  GotoTag=w_mc_out_r
  Goto Tag Visibility8 : GotoTagVisibility  GotoTag=bus_voltage_prev
  Goto Tag Visibility9 : GotoTagVisibility  GotoTag=v_prev
  help : Subsystem
      settings: OpenFcn=web(['file:\\\' which('motor_controller.htm')]);  RTWFcnNameOpts=Auto  RTWFileNameOpts=Auto
      mask Display: image(imread('doc_man.jpg'))
  mc model : Subsystem
      settings: RTWFcnNameOpts=Auto  RTWFileNameOpts=Auto
  signal annotator : Subsystem
      settings: RTWFcnNameOpts=Auto  RTWFileNameOpts=Auto
  Out Request : Outport  Port=1
  electric power in  requested : Outport  Port=2
  "trq and spd out achieved " : Outport  Port=3
  sensors : Outport  Port=4
  tag scope: bus_voltage_prev=scoped, current_veh_mass=scoped, cyc_mph_r_prev=scoped, key_on=scoped, mc_init_spd_est=scoped, mpha_prev=scoped, shifting=scoped, v_prev=scoped, veh_spd_a_rec_prev=scoped
  wires:
  [mc_max_crrnt] -> Bus Creator/7  "mc_max_crrnt"
  signal annotator/1(Out1) -> Out Request/1
  control/1 -> Demux/1
  Bus Creator/1 -> sensors/1
  Demux/7 -> [current_veh_mass]
  Demux/6 -> [cyc_mph_r_prev]
  [mc_spd_limited] -> Bus Creator/6  "mc_spd_limited"
  Demux/5 -> [mpha_prev]
  Demux/4 -> [bus_voltage_prev]
  Demux/3 -> [veh_spd_a_rec_prev]
  [w_mc_out_r] -> Bus Creator/5  "w_mc_out_r"
  [P_mc_in_1lim] -> Bus Creator/4  "P_mc_in_1lim"
  [mc_trq_limited] -> Bus Creator/3  "mc_trq_limited"
  [mc_spd_out_a] -> Bus Creator/2  "mc_spd_out_a"
  [mc_trq_out_a] -> Bus Creator/1  "mc_trq_out_a"
  Demux/2 -> [key_on]
  Demux/1 -> [v_prev]
  mc model/2("drive torque and speed avail. at rotor (Nm), (rad/s)") -> "trq and spd out achieved "/1
  mc model/1(req'd motor input power (W)) -> electric power in  requested/1
  electric power in achieved/1 -> mc model/2(available motor input power (W))
  trq and spd out requested/1 -> signal annotator/1(In1), mc model/1("torque and speed  req'd at rotor (Nm), (rad/s)")
  Demux/8 -> [shifting]
  [P_mc_in_r] -> Bus Creator/8  "P_mc_in_r"
  [mc_crrnt_limited] -> Bus Creator/9  "mc_crrnt_limited"
  Demux/9 -> [mc_init_spd_est]

== system bd_par_auto2/power bus <pb>/Block NOTES ==
  note: This block models the internal combustion engine, and includes inertia effects,
      | performance limits, accessory loads, and temperature transient effects on fuel
      | use, engine-out emissions, and catalyst efficiency.  There are 'leads' to the
      | engine controller here, which controller determines whether the engine is on.

== system bd_par_auto2/power bus <pb>/help ==

== system bd_par_auto2/power bus <pb>/power bus ==
  note: Power Bus Model
  note: Interface
  power out req : Inport  Port=1  LatchInput=off
  power available from source one : Inport  Port=2  LatchInput=off
  power available from source two : Inport  Port=3  LatchInput=off
  control : Inport  Port=4  LatchInput=off
  Demux : Demux  Outputs=1  BusSelectionMode=off
  Goto Tag Visibility : GotoTagVisibility  GotoTag=enable_source_two
  Ground : Ground
  model : Subsystem
      settings: RTWFcnNameOpts=Auto  RTWFileNameOpts=Auto
  signal annotator : Subsystem
      settings: RTWFcnNameOpts=Auto  RTWFileNameOpts=Auto
  required out : Outport  Port=1
  power in req from  source one : Outport  Port=2
  power in req from  source two : Outport  Port=3
  power out available : Outport  Port=4
  sensors : Outport  Port=5
  tag scope: enable_source_two=scoped
  wires:
  Ground/1 -> sensors/1
  Demux/1 -> [enable_source_two]
  control/1 -> Demux/1
  signal annotator/1(Out1) -> required out/1
  power available from source two/1 -> model/3(power available from energy storage (W))
  model/3(output power  available at bus) -> power out available/1
  power available from source one/1 -> model/2(power available from generator (W))
  model/2(power req'd from energy storage (W)) -> power in req from  source two/1
  power out req/1 -> signal annotator/1(In1), model/1(req'd power output (W))
  model/1(power req'd from generator (W)) -> power in req from  source one/1

== system bd_par_auto2/torque coupler <tc>/tc model & interface ==
  note: Model
  note: Interface
  trq and spd output request : Inport  Port=1  LatchInput=off
  trq and spd avail. at main input : Inport  Port=2  LatchInput=off
  trq and spd avail. at motor input to tc : Inport  Port=3  LatchInput=off
  controls : Inport  Port=4  LatchInput=off
  Ground : Ground
  Terminator : Terminator
  signal annotator : Subsystem
      settings: RTWFcnNameOpts=Auto  RTWFileNameOpts=Auto
  tc model : Subsystem
      settings: RTWFcnNameOpts=Auto  RTWFileNameOpts=Auto
  requested output : Outport  Port=1
  trq and spd req'd at main input : Outport  Port=2  InitialOutput=0
  trq and spd req'd at motor input to torque coupler : Outport  Port=3  InitialOutput=0
  trq and spd avail. at output side of torque coupler : Outport  Port=4  InitialOutput=0
  sensors : Outport  Port=5
  wires:
  Ground/1 -> sensors/1
  controls/1 -> Terminator/1
  signal annotator/1(Out1) -> requested output/1
  trq and spd output request/1 -> signal annotator/1(In1), tc model/1("torque and speed req'd at output side of torque coupler (Nm), (rad/s)")
  trq and spd avail. at motor input to tc/1 -> tc model/3("torque and speed avail. at motor input to tc (Nm), (rad/s)")
  tc model/3("torque and speed avail. at output side of torque coupler (Nm), (rad/s)") -> trq and spd avail. at output side of torque coupler/1
  trq and spd avail. at main input/1 -> tc model/2("torque and speed avail. at main input (Nm), (rad/s)")
  tc model/2("torque and speed req'd at motor input to torque coupler (Nm), (rad/s)") -> trq and spd req'd at motor input to torque coupler/1
  tc model/1("torque and speed req'd at main input to torque coupler (Nm), (rad/s)") -> trq and spd req'd at main input/1

== system bd_par_auto2/torque modification  strategy <cs>/Block NOTES ==
  note: This model allows for increasing or decreasing of torque along a connection for purposes
      | of hybrid charging and control strategy.

== system bd_par_auto2/torque modification  strategy <cs>/help1 ==

== system bd_par_auto2/torque modification  strategy <cs>/torque mod  model & interface ==
  note: Interface
  note: Model
  trq and spd output request : Inport  Port=1  LatchInput=off
  controls : Inport  Port=2  LatchInput=off
  Bus Creator : BusCreator  Inputs=4
  Demux2 : Demux  Outputs=3  BusSelectionMode=off
  Goto Tag Visibility1 : GotoTagVisibility  GotoTag=modifiedTorqueRequest
  Goto Tag Visibility2 : GotoTagVisibility  GotoTag=tm_torqueMod
  Goto Tag Visibility3 : GotoTagVisibility  GotoTag=tm_torqueMin
  Goto Tag Visibility4 : GotoTagVisibility  GotoTag=tm_enable
  model : Subsystem
      settings: RTWFcnNameOpts=Auto  RTWFileNameOpts=Auto
  signal annotator : Subsystem
      settings: RTWFcnNameOpts=Auto  RTWFileNameOpts=Auto
  requested output : Outport  Port=1
  trq and spd input request : Outport  Port=2
  sensors : Outport  Port=3
  tag scope: tm_enable=scoped, tm_torqueMin=scoped, tm_torqueMod=scoped
  wires:
  signal annotator/1(Out1) -> requested output/1
  model/1(T,w modified) -> trq and spd input request/1
  trq and spd output request/1 -> signal annotator/1(In1), model/1("T, w original")
  Demux2/1 -> [tm_torqueMod]
  controls/1 -> Demux2/1
  Bus Creator/1 -> sensors/1
  [tm_torqueMod] -> Bus Creator/1  "tm_torqueMod"
  Demux2/2 -> [tm_torqueMin]
  Demux2/3 -> [tm_enable]
  [tm_torqueMin] -> Bus Creator/2  "tm_torqueMin"
  [tm_enable] -> Bus Creator/3  "tm_enable"
  [modifiedTorqueRequest] -> Bus Creator/4  "modifiedTorqueRequest"
